simulink model "modelo_linear_pid"  (R2022a)
settings: Solver=VariableStepAuto  StartTime=0.0  StopTime=100  RelTol=1e-3
values from neighbouring files (symbols this model uses):
  A = [ 0 1 0  0 ... (first row only)    [ball_and_beam_pfc.m]
  amplitude_entrada = 0.05    [ball_and_beam_pfc.m]
  B = [0 ... (first row only)    [ball_and_beam_pfc.m]
  bool_degrau = 1    [ball_and_beam_pfc.m]
  C = [0 0 1 0]    [ball_and_beam_pfc.m]
  C2_A = [X(7) X(5) X(3) X(1)]    [ball_and_beam_pfc.m]
  C2_M = [X(8) X(6) X(4) X(2)]    [ball_and_beam_pfc.m]
  L = 0.425    [ball_and_beam_pfc.m]    (also in nonlinear_ball_and_beam.m)
  Ls = f(8)/a(5)    [ball_and_beam_pfc.m]
libraries: vrlib x3
settings Model: Creator=Notebook_Artur  LastModifiedBy=Notebook_Artur

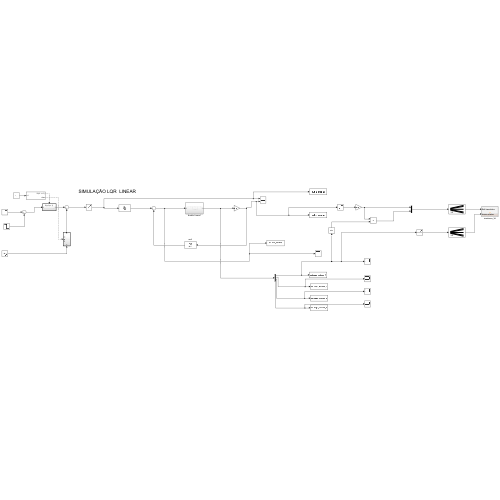
[thumbnail: Simulink's stored preview of the top-level diagram]
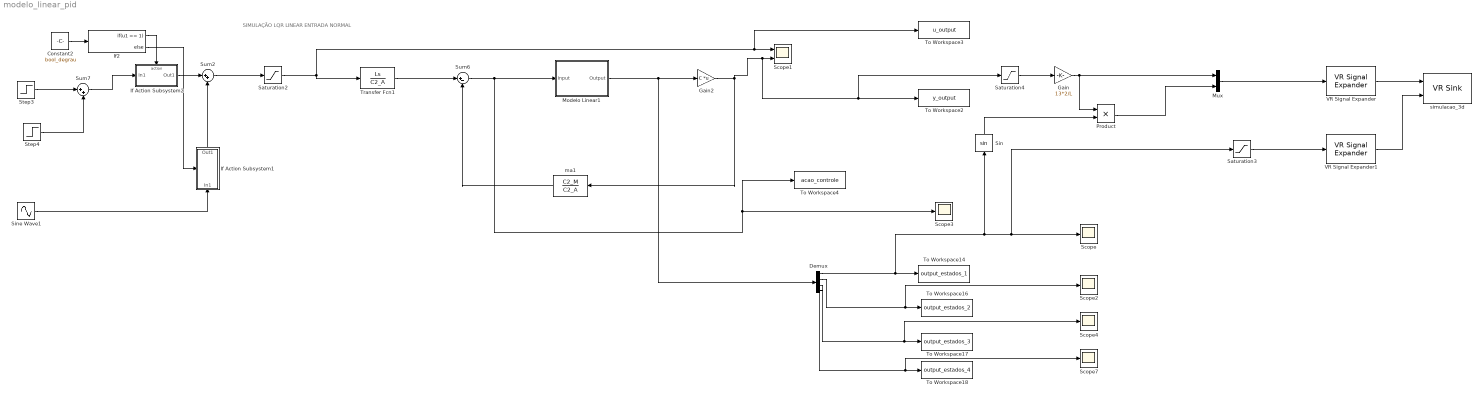
== system modelo_linear_pid ==
  note: SIMULAÇÃO LQR LINEAR ENTRADA NORMAL
  Constant2 : Constant  Value=bool_degrau
  Demux : Demux
  Gain : Gain  Gain=13*2/L
  Gain2 : Gain  Gain=C  Multiplication=Matrix(K*u)
  If Action Subsystem1 : Subsystem  TreatAsAtomicUnit=on
  If Action Subsystem2 : Subsystem  TreatAsAtomicUnit=on
  If2 : If  IfExpression=u1 == 1
  Modelo Linear1 : Subsystem
  Mux : Mux  Inputs=2
  Product : Product
  Saturation2 : Saturate  UpperLimit=L/2  LowerLimit=-L/2
  Saturation3 : Saturate  UpperLimit=0.1  LowerLimit=-0.1
  Saturation4 : Saturate  UpperLimit=L/2  LowerLimit=0
  Scope{,2..4,7} (5 alike) : Scope
  Scope1 : Scope  NumInputPorts=2
  Sin : Trigonometry
  Sine Wave1 : Sin  Amplitude=amplitude_entrada  Frequency=0.1  SampleTime=0
  Step3 : Step  After=amplitude_entrada  SampleTime=0
  Step4 : Step  Time=100  After=-2*amplitude_entrada  SampleTime=0
  Sum2 : Sum  Inputs=|++
  Sum6 : Sum  Inputs=|+-
  Sum7 : Sum  Inputs=|++
  To Workspace14 : ToWorkspace  VariableName=output_estados_1  SaveFormat=Timeseries  SampleTime=-1
  To Workspace16 : ToWorkspace  VariableName=output_estados_2  SaveFormat=Timeseries  SampleTime=-1
  To Workspace17 : ToWorkspace  VariableName=output_estados_3  SaveFormat=Timeseries  SampleTime=-1
  To Workspace18 : ToWorkspace  VariableName=output_estados_4  SaveFormat=Timeseries  SampleTime=-1
  To Workspace2 : ToWorkspace  VariableName=y_output  SaveFormat=Timeseries  SampleTime=-1
  To Workspace3 : ToWorkspace  VariableName=u_output  SaveFormat=Timeseries  SampleTime=-1
  To Workspace4 : ToWorkspace  VariableName=acao_controle  SaveFormat=Timeseries  SampleTime=-1
  Transfer Fcn1 : TransferFcn  Numerator=Ls  Denominator=C2_A
  VR Signal Expander : vrlib/VR Signal Expander  outwidth=3  outidx=[1 3]
  VR Signal Expander1 : vrlib/VR Signal Expander  outwidth=4  outidx=[4]
  ma1 : TransferFcn  Numerator=C2_M  Denominator=C2_A
  simulacao_3d : vrlib/VR Sink  InstantiateOnLoad=on  SampleTime=0.1  ViewEnable=on  RemoteChange=off  RemoteView=off  FieldsWritten=Ball.translation.3.1.1.double#beam.rotation.4.1.1.double  WorldFileName=3d_ball_and_beam4.x3d  AutoView=on  VideoDimensions=[]  AllowVariableSize=off
  wires:
  Gain/1 -> Product/1, Mux/1
  Sum7/1 -> If Action Subsystem2/1(In1)
  Modelo Linear1/1(Output) -> Demux/1, Gain2/1
  Mux/1 -> VR Signal Expander/1
  Sin/1 -> Product/2
  Step3/1 -> Sum7/1
  VR Signal Expander1/1 -> simulacao_3d/2
  Gain2/1 -> Saturation4/1, To Workspace2/1, Scope1/2, ma1/1
  Demux/1 -> Scope/1, Saturation3/1, Sin/1, To Workspace14/1
  Demux/2 -> Scope2/1, To Workspace16/1
  If2/1 -> If Action Subsystem2/Action
  Saturation3/1 -> VR Signal Expander1/1
  If Action Subsystem1/1(Out1) -> Sum2/2
  Product/1 -> Mux/2
  Constant2/1 -> If2/1
  Sum2/1 -> Saturation2/1
  Saturation2/1 -> To Workspace3/1, Scope1/1, Transfer Fcn1/1
  If2/2 -> If Action Subsystem1/Action
  Demux/3 -> Scope4/1, To Workspace17/1
  Sine Wave1/1 -> If Action Subsystem1/1(In1)
  If Action Subsystem2/1(Out1) -> Sum2/1
  Demux/4 -> Scope7/1, To Workspace18/1
  VR Signal Expander/1 -> simulacao_3d/1
  Saturation4/1 -> Gain/1
  Step4/1 -> Sum7/2
  Sum6/1 -> To Workspace4/1, Scope3/1, Modelo Linear1/1(Input)
  Transfer Fcn1/1 -> Sum6/1
  ma1/1 -> Sum6/2

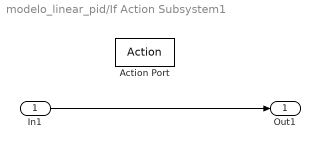
== system modelo_linear_pid/If Action Subsystem1 ==
  In1 : Inport
  Action Port : ActionPort  ActionPortLabel=else
  Out1 : Outport
  wires:
  In1/1 -> Out1/1

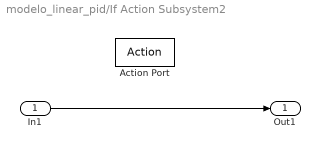
== system modelo_linear_pid/If Action Subsystem2 ==
  In1 : Inport
  Action Port : ActionPort  ActionPortLabel=if(u1 == 1)
  Out1 : Outport
  wires:
  In1/1 -> Out1/1

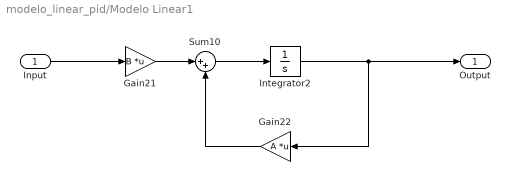
== system modelo_linear_pid/Modelo Linear1 ==
  Input : Inport
  Gain21 : Gain  Gain=B  Multiplication=Matrix(K*u)
  Gain22 : Gain  Gain=A  Multiplication=Matrix(K*u)
  Integrator2 : Integrator
  Sum10 : Sum  Inputs=|++
  Output : Outport
  wires:
  Input/1 -> Gain21/1
  Gain22/1 -> Sum10/2
  Integrator2/1 -> Output/1, Gain22/1
  Gain21/1 -> Sum10/1
  Sum10/1 -> Integrator2/1
